simulink model "snb_bx"  (R2012b)
settings: Solver=FixedStepDiscrete  SolverMode=SingleTasking  StartTime=0.0  StopTime=10000  RelTol=1e-3
undefined symbols (not defined in the file): Down, pfb_coeff_gen_calc, Up, xlipgetpartsetting
libraries: xbsIndex_r4 x14917, casper_library_misc x20, casper_library_communications x8, xps_library x3, casper_library_delays x3
(part 50 of 96)

== system snb_bx/mix_dec_fir/mixer/dds ==
  lo_const0 : Subsystem  AncestorBlock=casper_library_downconverter/lo_const  mask(lo_const){n_bits=10, phase=0}
      mask prompts: n_bits "Output Bitwidth"; phase "Phase (0 to 2*pi)"
      mask help:
      | Generates a complex constant associated with the
      | phase supplied as a parameter.
      mask init:
      | lo_const_init(gcb, ...
      |     'n_bits', n_bits, ...
      |     'phase', phase);
      mask Help: eval('xlWeb(''http://casper.berkeley.edu/wiki/Lo_const'')')
  lo_const1 : Subsystem  AncestorBlock=casper_library_downconverter/lo_const  mask(lo_const){n_bits=10, phase=1.5708}
      mask prompts: n_bits "Output Bitwidth"; phase "Phase (0 to 2*pi)"
      mask help:
      | Generates a complex constant associated with the
      | phase supplied as a parameter.
      mask init:
      | lo_const_init(gcb, ...
      |     'n_bits', n_bits, ...
      |     'phase', phase);
      mask Help: eval('xlWeb(''http://casper.berkeley.edu/wiki/Lo_const'')')
  lo_const2 : Subsystem  AncestorBlock=casper_library_downconverter/lo_const  mask(lo_const){n_bits=10, phase=3.1416}
      mask prompts: n_bits "Output Bitwidth"; phase "Phase (0 to 2*pi)"
      mask help:
      | Generates a complex constant associated with the
      | phase supplied as a parameter.
      mask init:
      | lo_const_init(gcb, ...
      |     'n_bits', n_bits, ...
      |     'phase', phase);
      mask Help: eval('xlWeb(''http://casper.berkeley.edu/wiki/Lo_const'')')
  lo_const3 : Subsystem  AncestorBlock=casper_library_downconverter/lo_const  mask(lo_const){n_bits=10, phase=4.7124}
      mask prompts: n_bits "Output Bitwidth"; phase "Phase (0 to 2*pi)"
      mask help:
      | Generates a complex constant associated with the
      | phase supplied as a parameter.
      mask init:
      | lo_const_init(gcb, ...
      |     'n_bits', n_bits, ...
      |     'phase', phase);
      mask Help: eval('xlWeb(''http://casper.berkeley.edu/wiki/Lo_const'')')
  lo_const4 : Subsystem  AncestorBlock=casper_library_downconverter/lo_const  mask(lo_const){n_bits=10, phase=6.2832}
      mask prompts: n_bits "Output Bitwidth"; phase "Phase (0 to 2*pi)"
      mask help:
      | Generates a complex constant associated with the
      | phase supplied as a parameter.
      mask init:
      | lo_const_init(gcb, ...
      |     'n_bits', n_bits, ...
      |     'phase', phase);
      mask Help: eval('xlWeb(''http://casper.berkeley.edu/wiki/Lo_const'')')
  lo_const5 : Subsystem  AncestorBlock=casper_library_downconverter/lo_const  mask(lo_const){n_bits=10, phase=7.854}
      mask prompts: n_bits "Output Bitwidth"; phase "Phase (0 to 2*pi)"
      mask help:
      | Generates a complex constant associated with the
      | phase supplied as a parameter.
      mask init:
      | lo_const_init(gcb, ...
      |     'n_bits', n_bits, ...
      |     'phase', phase);
      mask Help: eval('xlWeb(''http://casper.berkeley.edu/wiki/Lo_const'')')
  lo_const6 : Subsystem  AncestorBlock=casper_library_downconverter/lo_const  mask(lo_const){n_bits=10, phase=9.4248}
      mask prompts: n_bits "Output Bitwidth"; phase "Phase (0 to 2*pi)"
      mask help:
      | Generates a complex constant associated with the
      | phase supplied as a parameter.
      mask init:
      | lo_const_init(gcb, ...
      |     'n_bits', n_bits, ...
      |     'phase', phase);
      mask Help: eval('xlWeb(''http://casper.berkeley.edu/wiki/Lo_const'')')
  lo_const7 : Subsystem  AncestorBlock=casper_library_downconverter/lo_const  mask(lo_const){n_bits=10, phase=10.9956}
      mask prompts: n_bits "Output Bitwidth"; phase "Phase (0 to 2*pi)"
      mask help:
      | Generates a complex constant associated with the
      | phase supplied as a parameter.
      mask init:
      | lo_const_init(gcb, ...
      |     'n_bits', n_bits, ...
      |     'phase', phase);
      mask Help: eval('xlWeb(''http://casper.berkeley.edu/wiki/Lo_const'')')
  sin0 : Outport
  cos0 : Outport  Port=2
  sin1 : Outport  Port=3
  cos1 : Outport  Port=4
  sin2 : Outport  Port=5
  cos2 : Outport  Port=6
  sin3 : Outport  Port=7
  cos3 : Outport  Port=8
  sin4 : Outport  Port=9
  cos4 : Outport  Port=10
  sin5 : Outport  Port=11
  cos5 : Outport  Port=12
  sin6 : Outport  Port=13
  cos6 : Outport  Port=14
  sin7 : Outport  Port=15
  cos7 : Outport  Port=16
  wires:
  lo_const0/1(sin) -> sin0/1
  lo_const0/2(cos) -> cos0/1
  lo_const1/1(sin) -> sin1/1
  lo_const1/2(cos) -> cos1/1
  lo_const2/1(sin) -> sin2/1
  lo_const2/2(cos) -> cos2/1
  lo_const3/1(sin) -> sin3/1
  lo_const3/2(cos) -> cos3/1
  lo_const4/1(sin) -> sin4/1
  lo_const4/2(cos) -> cos4/1
  lo_const5/1(sin) -> sin5/1
  lo_const5/2(cos) -> cos5/1
  lo_const6/1(sin) -> sin6/1
  lo_const6/2(cos) -> cos6/1
  lo_const7/1(sin) -> sin7/1
  lo_const7/2(cos) -> cos7/1

== system snb_bx/mix_dec_fir/mixer/rcmult1 ==
  d : Inport
  sin : Inport  Port=2
  cos : Inport  Port=3
  Mult0 : xbsIndex_r4/Mult  precision=Full  arith_type="Signed  (2's comp)"  n_bits=8  bin_pt=2  quantization=Truncate  overflow=Wrap  en=off  latency=latency  dbl_ovrd=off  use_behavioral_HDL=off  opt=Speed  use_embedded=on  optimum_pipeline=off  pipeline=on  use_rpm=off  placement_style=Rectangular shape  block_type=mult
  Mult1 : xbsIndex_r4/Mult  precision=Full  arith_type="Signed  (2's comp)"  n_bits=8  bin_pt=2  quantization=Truncate  overflow=Wrap  en=off  latency=latency  dbl_ovrd=off  use_behavioral_HDL=off  opt=Speed  use_embedded=on  optimum_pipeline=off  pipeline=on  use_rpm=off  placement_style=Rectangular shape  block_type=mult
  real : Outport
  imag : Outport  Port=2
  wires:
  cos/1 -> Mult0/2
  sin/1 -> Mult1/2
  d/1 -> Mult1/1, Mult0/1
  Mult0/1 -> real/1
  Mult1/1 -> imag/1

== system snb_bx/mix_dec_fir/mixer/rcmult2 ==
  d : Inport
  sin : Inport  Port=2
  cos : Inport  Port=3
  Mult0 : xbsIndex_r4/Mult  precision=Full  arith_type="Signed  (2's comp)"  n_bits=8  bin_pt=2  quantization=Truncate  overflow=Wrap  en=off  latency=latency  dbl_ovrd=off  use_behavioral_HDL=off  opt=Speed  use_embedded=on  optimum_pipeline=off  pipeline=on  use_rpm=off  placement_style=Rectangular shape  block_type=mult
  Mult1 : xbsIndex_r4/Mult  precision=Full  arith_type="Signed  (2's comp)"  n_bits=8  bin_pt=2  quantization=Truncate  overflow=Wrap  en=off  latency=latency  dbl_ovrd=off  use_behavioral_HDL=off  opt=Speed  use_embedded=on  optimum_pipeline=off  pipeline=on  use_rpm=off  placement_style=Rectangular shape  block_type=mult
  real : Outport
  imag : Outport  Port=2
  wires:
  cos/1 -> Mult0/2
  sin/1 -> Mult1/2
  d/1 -> Mult1/1, Mult0/1
  Mult0/1 -> real/1
  Mult1/1 -> imag/1

== system snb_bx/mix_dec_fir/mixer/rcmult3 ==
  d : Inport
  sin : Inport  Port=2
  cos : Inport  Port=3
  Mult0 : xbsIndex_r4/Mult  precision=Full  arith_type="Signed  (2's comp)"  n_bits=8  bin_pt=2  quantization=Truncate  overflow=Wrap  en=off  latency=latency  dbl_ovrd=off  use_behavioral_HDL=off  opt=Speed  use_embedded=on  optimum_pipeline=off  pipeline=on  use_rpm=off  placement_style=Rectangular shape  block_type=mult
  Mult1 : xbsIndex_r4/Mult  precision=Full  arith_type="Signed  (2's comp)"  n_bits=8  bin_pt=2  quantization=Truncate  overflow=Wrap  en=off  latency=latency  dbl_ovrd=off  use_behavioral_HDL=off  opt=Speed  use_embedded=on  optimum_pipeline=off  pipeline=on  use_rpm=off  placement_style=Rectangular shape  block_type=mult
  real : Outport
  imag : Outport  Port=2
  wires:
  cos/1 -> Mult0/2
  sin/1 -> Mult1/2
  d/1 -> Mult1/1, Mult0/1
  Mult0/1 -> real/1
  Mult1/1 -> imag/1

== system snb_bx/mix_dec_fir/mixer/rcmult4 ==
  d : Inport
  sin : Inport  Port=2
  cos : Inport  Port=3
  Mult0 : xbsIndex_r4/Mult  precision=Full  arith_type="Signed  (2's comp)"  n_bits=8  bin_pt=2  quantization=Truncate  overflow=Wrap  en=off  latency=latency  dbl_ovrd=off  use_behavioral_HDL=off  opt=Speed  use_embedded=on  optimum_pipeline=off  pipeline=on  use_rpm=off  placement_style=Rectangular shape  block_type=mult
  Mult1 : xbsIndex_r4/Mult  precision=Full  arith_type="Signed  (2's comp)"  n_bits=8  bin_pt=2  quantization=Truncate  overflow=Wrap  en=off  latency=latency  dbl_ovrd=off  use_behavioral_HDL=off  opt=Speed  use_embedded=on  optimum_pipeline=off  pipeline=on  use_rpm=off  placement_style=Rectangular shape  block_type=mult
  real : Outport
  imag : Outport  Port=2
  wires:
  cos/1 -> Mult0/2
  sin/1 -> Mult1/2
  d/1 -> Mult1/1, Mult0/1
  Mult0/1 -> real/1
  Mult1/1 -> imag/1

== system snb_bx/mix_dec_fir/mixer/rcmult5 ==
  d : Inport
  sin : Inport  Port=2
  cos : Inport  Port=3
  Mult0 : xbsIndex_r4/Mult  precision=Full  arith_type="Signed  (2's comp)"  n_bits=8  bin_pt=2  quantization=Truncate  overflow=Wrap  en=off  latency=latency  dbl_ovrd=off  use_behavioral_HDL=off  opt=Speed  use_embedded=on  optimum_pipeline=off  pipeline=on  use_rpm=off  placement_style=Rectangular shape  block_type=mult
  Mult1 : xbsIndex_r4/Mult  precision=Full  arith_type="Signed  (2's comp)"  n_bits=8  bin_pt=2  quantization=Truncate  overflow=Wrap  en=off  latency=latency  dbl_ovrd=off  use_behavioral_HDL=off  opt=Speed  use_embedded=on  optimum_pipeline=off  pipeline=on  use_rpm=off  placement_style=Rectangular shape  block_type=mult
  real : Outport
  imag : Outport  Port=2
  wires:
  cos/1 -> Mult0/2
  sin/1 -> Mult1/2
  d/1 -> Mult1/1, Mult0/1
  Mult0/1 -> real/1
  Mult1/1 -> imag/1

== system snb_bx/mix_dec_fir/mixer/rcmult6 ==
  d : Inport
  sin : Inport  Port=2
  cos : Inport  Port=3
  Mult0 : xbsIndex_r4/Mult  precision=Full  arith_type="Signed  (2's comp)"  n_bits=8  bin_pt=2  quantization=Truncate  overflow=Wrap  en=off  latency=latency  dbl_ovrd=off  use_behavioral_HDL=off  opt=Speed  use_embedded=on  optimum_pipeline=off  pipeline=on  use_rpm=off  placement_style=Rectangular shape  block_type=mult
  Mult1 : xbsIndex_r4/Mult  precision=Full  arith_type="Signed  (2's comp)"  n_bits=8  bin_pt=2  quantization=Truncate  overflow=Wrap  en=off  latency=latency  dbl_ovrd=off  use_behavioral_HDL=off  opt=Speed  use_embedded=on  optimum_pipeline=off  pipeline=on  use_rpm=off  placement_style=Rectangular shape  block_type=mult
  real : Outport
  imag : Outport  Port=2
  wires:
  cos/1 -> Mult0/2
  sin/1 -> Mult1/2
  d/1 -> Mult1/1, Mult0/1
  Mult0/1 -> real/1
  Mult1/1 -> imag/1

== system snb_bx/mix_dec_fir/mixer/rcmult7 ==
  d : Inport
  sin : Inport  Port=2
  cos : Inport  Port=3
  Mult0 : xbsIndex_r4/Mult  precision=Full  arith_type="Signed  (2's comp)"  n_bits=8  bin_pt=2  quantization=Truncate  overflow=Wrap  en=off  latency=latency  dbl_ovrd=off  use_behavioral_HDL=off  opt=Speed  use_embedded=on  optimum_pipeline=off  pipeline=on  use_rpm=off  placement_style=Rectangular shape  block_type=mult
  Mult1 : xbsIndex_r4/Mult  precision=Full  arith_type="Signed  (2's comp)"  n_bits=8  bin_pt=2  quantization=Truncate  overflow=Wrap  en=off  latency=latency  dbl_ovrd=off  use_behavioral_HDL=off  opt=Speed  use_embedded=on  optimum_pipeline=off  pipeline=on  use_rpm=off  placement_style=Rectangular shape  block_type=mult
  real : Outport
  imag : Outport  Port=2
  wires:
  cos/1 -> Mult0/2
  sin/1 -> Mult1/2
  d/1 -> Mult1/1, Mult0/1
  Mult0/1 -> real/1
  Mult1/1 -> imag/1

== system snb_bx/mix_dec_fir/mixer/rcmult8 ==
  d : Inport
  sin : Inport  Port=2
  cos : Inport  Port=3
  Mult0 : xbsIndex_r4/Mult  precision=Full  arith_type="Signed  (2's comp)"  n_bits=8  bin_pt=2  quantization=Truncate  overflow=Wrap  en=off  latency=latency  dbl_ovrd=off  use_behavioral_HDL=off  opt=Speed  use_embedded=on  optimum_pipeline=off  pipeline=on  use_rpm=off  placement_style=Rectangular shape  block_type=mult
  Mult1 : xbsIndex_r4/Mult  precision=Full  arith_type="Signed  (2's comp)"  n_bits=8  bin_pt=2  quantization=Truncate  overflow=Wrap  en=off  latency=latency  dbl_ovrd=off  use_behavioral_HDL=off  opt=Speed  use_embedded=on  optimum_pipeline=off  pipeline=on  use_rpm=off  placement_style=Rectangular shape  block_type=mult
  real : Outport
  imag : Outport  Port=2
  wires:
  cos/1 -> Mult0/2
  sin/1 -> Mult1/2
  d/1 -> Mult1/1, Mult0/1
  Mult0/1 -> real/1
  Mult1/1 -> imag/1

== system snb_bx/mix_dec_fir/mixer1/dds ==
  lo_const0 : Subsystem  AncestorBlock=casper_library_downconverter/lo_const  mask(lo_const){n_bits=10, phase=0}
      mask prompts: n_bits "Output Bitwidth"; phase "Phase (0 to 2*pi)"
      mask help:
      | Generates a complex constant associated with the
      | phase supplied as a parameter.
      mask init:
      | lo_const_init(gcb, ...
      |     'n_bits', n_bits, ...
      |     'phase', phase);
      mask Help: eval('xlWeb(''http://casper.berkeley.edu/wiki/Lo_const'')')
  lo_const1 : Subsystem  AncestorBlock=casper_library_downconverter/lo_const  mask(lo_const){n_bits=10, phase=1.5708}
      mask prompts: n_bits "Output Bitwidth"; phase "Phase (0 to 2*pi)"
      mask help:
      | Generates a complex constant associated with the
      | phase supplied as a parameter.
      mask init:
      | lo_const_init(gcb, ...
      |     'n_bits', n_bits, ...
      |     'phase', phase);
      mask Help: eval('xlWeb(''http://casper.berkeley.edu/wiki/Lo_const'')')
  lo_const2 : Subsystem  AncestorBlock=casper_library_downconverter/lo_const  mask(lo_const){n_bits=10, phase=3.1416}
      mask prompts: n_bits "Output Bitwidth"; phase "Phase (0 to 2*pi)"
      mask help:
      | Generates a complex constant associated with the
      | phase supplied as a parameter.
      mask init:
      | lo_const_init(gcb, ...
      |     'n_bits', n_bits, ...
      |     'phase', phase);
      mask Help: eval('xlWeb(''http://casper.berkeley.edu/wiki/Lo_const'')')
  lo_const3 : Subsystem  AncestorBlock=casper_library_downconverter/lo_const  mask(lo_const){n_bits=10, phase=4.7124}
      mask prompts: n_bits "Output Bitwidth"; phase "Phase (0 to 2*pi)"
      mask help:
      | Generates a complex constant associated with the
      | phase supplied as a parameter.
      mask init:
      | lo_const_init(gcb, ...
      |     'n_bits', n_bits, ...
      |     'phase', phase);
      mask Help: eval('xlWeb(''http://casper.berkeley.edu/wiki/Lo_const'')')
  lo_const4 : Subsystem  AncestorBlock=casper_library_downconverter/lo_const  mask(lo_const){n_bits=10, phase=6.2832}
      mask prompts: n_bits "Output Bitwidth"; phase "Phase (0 to 2*pi)"
      mask help:
      | Generates a complex constant associated with the
      | phase supplied as a parameter.
      mask init:
      | lo_const_init(gcb, ...
      |     'n_bits', n_bits, ...
      |     'phase', phase);
      mask Help: eval('xlWeb(''http://casper.berkeley.edu/wiki/Lo_const'')')
  lo_const5 : Subsystem  AncestorBlock=casper_library_downconverter/lo_const  mask(lo_const){n_bits=10, phase=7.854}
      mask prompts: n_bits "Output Bitwidth"; phase "Phase (0 to 2*pi)"
      mask help:
      | Generates a complex constant associated with the
      | phase supplied as a parameter.
      mask init:
      | lo_const_init(gcb, ...
      |     'n_bits', n_bits, ...
      |     'phase', phase);
      mask Help: eval('xlWeb(''http://casper.berkeley.edu/wiki/Lo_const'')')
  lo_const6 : Subsystem  AncestorBlock=casper_library_downconverter/lo_const  mask(lo_const){n_bits=10, phase=9.4248}
      mask prompts: n_bits "Output Bitwidth"; phase "Phase (0 to 2*pi)"
      mask help:
      | Generates a complex constant associated with the
      | phase supplied as a parameter.
      mask init:
      | lo_const_init(gcb, ...
      |     'n_bits', n_bits, ...
      |     'phase', phase);
      mask Help: eval('xlWeb(''http://casper.berkeley.edu/wiki/Lo_const'')')
  lo_const7 : Subsystem  AncestorBlock=casper_library_downconverter/lo_const  mask(lo_const){n_bits=10, phase=10.9956}
      mask prompts: n_bits "Output Bitwidth"; phase "Phase (0 to 2*pi)"
      mask help:
      | Generates a complex constant associated with the
      | phase supplied as a parameter.
      mask init:
      | lo_const_init(gcb, ...
      |     'n_bits', n_bits, ...
      |     'phase', phase);
      mask Help: eval('xlWeb(''http://casper.berkeley.edu/wiki/Lo_const'')')
  sin0 : Outport
  cos0 : Outport  Port=2
  sin1 : Outport  Port=3
  cos1 : Outport  Port=4
  sin2 : Outport  Port=5
  cos2 : Outport  Port=6
  sin3 : Outport  Port=7
  cos3 : Outport  Port=8
  sin4 : Outport  Port=9
  cos4 : Outport  Port=10
  sin5 : Outport  Port=11
  cos5 : Outport  Port=12
  sin6 : Outport  Port=13
  cos6 : Outport  Port=14
  sin7 : Outport  Port=15
  cos7 : Outport  Port=16
  wires:
  lo_const7/2(cos) -> cos7/1
  lo_const7/1(sin) -> sin7/1
  lo_const6/2(cos) -> cos6/1
  lo_const6/1(sin) -> sin6/1
  lo_const5/2(cos) -> cos5/1
  lo_const5/1(sin) -> sin5/1
  lo_const4/2(cos) -> cos4/1
  lo_const4/1(sin) -> sin4/1
  lo_const3/2(cos) -> cos3/1
  lo_const3/1(sin) -> sin3/1
  lo_const2/2(cos) -> cos2/1
  lo_const2/1(sin) -> sin2/1
  lo_const1/2(cos) -> cos1/1
  lo_const1/1(sin) -> sin1/1
  lo_const0/2(cos) -> cos0/1
  lo_const0/1(sin) -> sin0/1

== system snb_bx/mix_dec_fir/mixer1/rcmult1 ==
  d : Inport
  sin : Inport  Port=2
  cos : Inport  Port=3
  Mult0 : xbsIndex_r4/Mult  precision=Full  arith_type="Signed  (2's comp)"  n_bits=8  bin_pt=2  quantization=Truncate  overflow=Wrap  en=off  latency=latency  dbl_ovrd=off  use_behavioral_HDL=off  opt=Speed  use_embedded=on  optimum_pipeline=off  pipeline=on  use_rpm=off  placement_style=Rectangular shape  block_type=mult
  Mult1 : xbsIndex_r4/Mult  precision=Full  arith_type="Signed  (2's comp)"  n_bits=8  bin_pt=2  quantization=Truncate  overflow=Wrap  en=off  latency=latency  dbl_ovrd=off  use_behavioral_HDL=off  opt=Speed  use_embedded=on  optimum_pipeline=off  pipeline=on  use_rpm=off  placement_style=Rectangular shape  block_type=mult
  real : Outport
  imag : Outport  Port=2
  wires:
  Mult1/1 -> imag/1
  Mult0/1 -> real/1
  d/1 -> Mult0/1, Mult1/1
  sin/1 -> Mult1/2
  cos/1 -> Mult0/2

== system snb_bx/mix_dec_fir/mixer1/rcmult2 ==
  d : Inport
  sin : Inport  Port=2
  cos : Inport  Port=3
  Mult0 : xbsIndex_r4/Mult  precision=Full  arith_type="Signed  (2's comp)"  n_bits=8  bin_pt=2  quantization=Truncate  overflow=Wrap  en=off  latency=latency  dbl_ovrd=off  use_behavioral_HDL=off  opt=Speed  use_embedded=on  optimum_pipeline=off  pipeline=on  use_rpm=off  placement_style=Rectangular shape  block_type=mult
  Mult1 : xbsIndex_r4/Mult  precision=Full  arith_type="Signed  (2's comp)"  n_bits=8  bin_pt=2  quantization=Truncate  overflow=Wrap  en=off  latency=latency  dbl_ovrd=off  use_behavioral_HDL=off  opt=Speed  use_embedded=on  optimum_pipeline=off  pipeline=on  use_rpm=off  placement_style=Rectangular shape  block_type=mult
  real : Outport
  imag : Outport  Port=2
  wires:
  Mult1/1 -> imag/1
  Mult0/1 -> real/1
  d/1 -> Mult0/1, Mult1/1
  sin/1 -> Mult1/2
  cos/1 -> Mult0/2

== system snb_bx/mix_dec_fir/mixer1/rcmult3 ==
  d : Inport
  sin : Inport  Port=2
  cos : Inport  Port=3
  Mult0 : xbsIndex_r4/Mult  precision=Full  arith_type="Signed  (2's comp)"  n_bits=8  bin_pt=2  quantization=Truncate  overflow=Wrap  en=off  latency=latency  dbl_ovrd=off  use_behavioral_HDL=off  opt=Speed  use_embedded=on  optimum_pipeline=off  pipeline=on  use_rpm=off  placement_style=Rectangular shape  block_type=mult
  Mult1 : xbsIndex_r4/Mult  precision=Full  arith_type="Signed  (2's comp)"  n_bits=8  bin_pt=2  quantization=Truncate  overflow=Wrap  en=off  latency=latency  dbl_ovrd=off  use_behavioral_HDL=off  opt=Speed  use_embedded=on  optimum_pipeline=off  pipeline=on  use_rpm=off  placement_style=Rectangular shape  block_type=mult
  real : Outport
  imag : Outport  Port=2
  wires:
  Mult1/1 -> imag/1
  Mult0/1 -> real/1
  d/1 -> Mult0/1, Mult1/1
  sin/1 -> Mult1/2
  cos/1 -> Mult0/2

== system snb_bx/mix_dec_fir/mixer1/rcmult4 ==
  d : Inport
  sin : Inport  Port=2
  cos : Inport  Port=3
  Mult0 : xbsIndex_r4/Mult  precision=Full  arith_type="Signed  (2's comp)"  n_bits=8  bin_pt=2  quantization=Truncate  overflow=Wrap  en=off  latency=latency  dbl_ovrd=off  use_behavioral_HDL=off  opt=Speed  use_embedded=on  optimum_pipeline=off  pipeline=on  use_rpm=off  placement_style=Rectangular shape  block_type=mult
  Mult1 : xbsIndex_r4/Mult  precision=Full  arith_type="Signed  (2's comp)"  n_bits=8  bin_pt=2  quantization=Truncate  overflow=Wrap  en=off  latency=latency  dbl_ovrd=off  use_behavioral_HDL=off  opt=Speed  use_embedded=on  optimum_pipeline=off  pipeline=on  use_rpm=off  placement_style=Rectangular shape  block_type=mult
  real : Outport
  imag : Outport  Port=2
  wires:
  Mult1/1 -> imag/1
  Mult0/1 -> real/1
  d/1 -> Mult0/1, Mult1/1
  sin/1 -> Mult1/2
  cos/1 -> Mult0/2

== system snb_bx/mix_dec_fir/mixer1/rcmult5 ==
  d : Inport
  sin : Inport  Port=2
  cos : Inport  Port=3
  Mult0 : xbsIndex_r4/Mult  precision=Full  arith_type="Signed  (2's comp)"  n_bits=8  bin_pt=2  quantization=Truncate  overflow=Wrap  en=off  latency=latency  dbl_ovrd=off  use_behavioral_HDL=off  opt=Speed  use_embedded=on  optimum_pipeline=off  pipeline=on  use_rpm=off  placement_style=Rectangular shape  block_type=mult
  Mult1 : xbsIndex_r4/Mult  precision=Full  arith_type="Signed  (2's comp)"  n_bits=8  bin_pt=2  quantization=Truncate  overflow=Wrap  en=off  latency=latency  dbl_ovrd=off  use_behavioral_HDL=off  opt=Speed  use_embedded=on  optimum_pipeline=off  pipeline=on  use_rpm=off  placement_style=Rectangular shape  block_type=mult
  real : Outport
  imag : Outport  Port=2
  wires:
  Mult1/1 -> imag/1
  Mult0/1 -> real/1
  d/1 -> Mult0/1, Mult1/1
  sin/1 -> Mult1/2
  cos/1 -> Mult0/2

== system snb_bx/mix_dec_fir/mixer1/rcmult6 ==
  d : Inport
  sin : Inport  Port=2
  cos : Inport  Port=3
  Mult0 : xbsIndex_r4/Mult  precision=Full  arith_type="Signed  (2's comp)"  n_bits=8  bin_pt=2  quantization=Truncate  overflow=Wrap  en=off  latency=latency  dbl_ovrd=off  use_behavioral_HDL=off  opt=Speed  use_embedded=on  optimum_pipeline=off  pipeline=on  use_rpm=off  placement_style=Rectangular shape  block_type=mult
  Mult1 : xbsIndex_r4/Mult  precision=Full  arith_type="Signed  (2's comp)"  n_bits=8  bin_pt=2  quantization=Truncate  overflow=Wrap  en=off  latency=latency  dbl_ovrd=off  use_behavioral_HDL=off  opt=Speed  use_embedded=on  optimum_pipeline=off  pipeline=on  use_rpm=off  placement_style=Rectangular shape  block_type=mult
  real : Outport
  imag : Outport  Port=2
  wires:
  Mult1/1 -> imag/1
  Mult0/1 -> real/1
  d/1 -> Mult0/1, Mult1/1
  sin/1 -> Mult1/2
  cos/1 -> Mult0/2

== system snb_bx/mix_dec_fir/mixer1/rcmult7 ==
  d : Inport
  sin : Inport  Port=2
  cos : Inport  Port=3
  Mult0 : xbsIndex_r4/Mult  precision=Full  arith_type="Signed  (2's comp)"  n_bits=8  bin_pt=2  quantization=Truncate  overflow=Wrap  en=off  latency=latency  dbl_ovrd=off  use_behavioral_HDL=off  opt=Speed  use_embedded=on  optimum_pipeline=off  pipeline=on  use_rpm=off  placement_style=Rectangular shape  block_type=mult
  Mult1 : xbsIndex_r4/Mult  precision=Full  arith_type="Signed  (2's comp)"  n_bits=8  bin_pt=2  quantization=Truncate  overflow=Wrap  en=off  latency=latency  dbl_ovrd=off  use_behavioral_HDL=off  opt=Speed  use_embedded=on  optimum_pipeline=off  pipeline=on  use_rpm=off  placement_style=Rectangular shape  block_type=mult
  real : Outport
  imag : Outport  Port=2
  wires:
  Mult1/1 -> imag/1
  Mult0/1 -> real/1
  d/1 -> Mult0/1, Mult1/1
  sin/1 -> Mult1/2
  cos/1 -> Mult0/2

== system snb_bx/mix_dec_fir/mixer1/rcmult8 ==
  d : Inport
  sin : Inport  Port=2
  cos : Inport  Port=3
  Mult0 : xbsIndex_r4/Mult  precision=Full  arith_type="Signed  (2's comp)"  n_bits=8  bin_pt=2  quantization=Truncate  overflow=Wrap  en=off  latency=latency  dbl_ovrd=off  use_behavioral_HDL=off  opt=Speed  use_embedded=on  optimum_pipeline=off  pipeline=on  use_rpm=off  placement_style=Rectangular shape  block_type=mult
  Mult1 : xbsIndex_r4/Mult  precision=Full  arith_type="Signed  (2's comp)"  n_bits=8  bin_pt=2  quantization=Truncate  overflow=Wrap  en=off  latency=latency  dbl_ovrd=off  use_behavioral_HDL=off  opt=Speed  use_embedded=on  optimum_pipeline=off  pipeline=on  use_rpm=off  placement_style=Rectangular shape  block_type=mult
  real : Outport
  imag : Outport  Port=2
  wires:
  Mult1/1 -> imag/1
  Mult0/1 -> real/1
  d/1 -> Mult0/1, Mult1/1
  sin/1 -> Mult1/2
  cos/1 -> Mult0/2

== system snb_bx/pack/spead_pack/edge_detect1 ==
  in : Inport
  Delay : xbsIndex_r4/Delay  rst=off  infoeditControl=Selection of Reset will increase slice count due to use of real FFs and instead of SRLs  en=off  latency=1  dbl_ovrd=off  reg_retiming=off  block_type=delay
      settings: xl_area=[0, 0, 0, 0, 0, 0, 0]
  Inverter : xbsIndex_r4/Inverter  en=off  latency=0  dbl_ovrd=off  block_type=inv
      settings: xl_area=[0, 0, 0, 0, 0, 0, 0]
  edge_op : xbsIndex_r4/Logical  logical_function=NOR  inputs=2  en=off  latency=0  precision=Full  arith_type=Unsigned  n_bits=8  bin_pt=2  align_bp=on  dbl_ovrd=off  block_type=logical
      settings: xl_area=[0, 0, 0, 0, 0, 0, 0]
  out : Outport
  wires:
  Delay/1 -> edge_op/2
  in/1 -> Delay/1, Inverter/1
  edge_op/1 -> out/1
  Inverter/1 -> edge_op/1

== system snb_bx/pack/spead_pack/edge_detect2 ==
  in : Inport
  Delay : xbsIndex_r4/Delay  rst=off  infoeditControl=Selection of Reset will increase slice count due to use of real FFs and instead of SRLs  en=off  latency=1  dbl_ovrd=off  reg_retiming=off  block_type=delay
      settings: xl_area=[0, 0, 0, 0, 0, 0, 0]
  Inverter : xbsIndex_r4/Inverter  en=off  latency=0  dbl_ovrd=off  block_type=inv
      settings: xl_area=[0, 0, 0, 0, 0, 0, 0]
  edge_op : xbsIndex_r4/Logical  logical_function=NOR  inputs=2  en=off  latency=0  precision=Full  arith_type=Unsigned  n_bits=8  bin_pt=2  align_bp=on  dbl_ovrd=off  block_type=logical
      settings: xl_area=[0, 0, 0, 0, 0, 0, 0]
  out : Outport
  wires:
  Inverter/1 -> edge_op/1
  edge_op/1 -> out/1
  in/1 -> Inverter/1, Delay/1
  Delay/1 -> edge_op/2

== system snb_bx/pack/spead_pack1/edge_detect1 ==
  in : Inport
  Delay : xbsIndex_r4/Delay  rst=off  infoeditControl=Selection of Reset will increase slice count due to use of real FFs and instead of SRLs  en=off  latency=1  dbl_ovrd=off  reg_retiming=off  block_type=delay
      settings: xl_area=[0, 0, 0, 0, 0, 0, 0]
  Inverter : xbsIndex_r4/Inverter  en=off  latency=0  dbl_ovrd=off  block_type=inv
      settings: xl_area=[0, 0, 0, 0, 0, 0, 0]
  edge_op : xbsIndex_r4/Logical  logical_function=NOR  inputs=2  en=off  latency=0  precision=Full  arith_type=Unsigned  n_bits=8  bin_pt=2  align_bp=on  dbl_ovrd=off  block_type=logical
      settings: xl_area=[0, 0, 0, 0, 0, 0, 0]
  out : Outport
  wires:
  Inverter/1 -> edge_op/1
  edge_op/1 -> out/1
  in/1 -> Inverter/1, Delay/1
  Delay/1 -> edge_op/2

== system snb_bx/pack/spead_pack1/edge_detect2 ==
  in : Inport
  Delay : xbsIndex_r4/Delay  rst=off  infoeditControl=Selection of Reset will increase slice count due to use of real FFs and instead of SRLs  en=off  latency=1  dbl_ovrd=off  reg_retiming=off  block_type=delay
      settings: xl_area=[0, 0, 0, 0, 0, 0, 0]
  Inverter : xbsIndex_r4/Inverter  en=off  latency=0  dbl_ovrd=off  block_type=inv
      settings: xl_area=[0, 0, 0, 0, 0, 0, 0]
  edge_op : xbsIndex_r4/Logical  logical_function=NOR  inputs=2  en=off  latency=0  precision=Full  arith_type=Unsigned  n_bits=8  bin_pt=2  align_bp=on  dbl_ovrd=off  block_type=logical
      settings: xl_area=[0, 0, 0, 0, 0, 0, 0]
  out : Outport
  wires:
  Delay/1 -> edge_op/2
  in/1 -> Delay/1, Inverter/1
  edge_op/1 -> out/1
  Inverter/1 -> edge_op/1

== system snb_bx/pack/spead_pack2/edge_detect1 ==
  in : Inport
  Delay : xbsIndex_r4/Delay  rst=off  infoeditControl=Selection of Reset will increase slice count due to use of real FFs and instead of SRLs  en=off  latency=1  dbl_ovrd=off  reg_retiming=off  block_type=delay
      settings: xl_area=[0, 0, 0, 0, 0, 0, 0]
  Inverter : xbsIndex_r4/Inverter  en=off  latency=0  dbl_ovrd=off  block_type=inv
      settings: xl_area=[0, 0, 0, 0, 0, 0, 0]
  edge_op : xbsIndex_r4/Logical  logical_function=NOR  inputs=2  en=off  latency=0  precision=Full  arith_type=Unsigned  n_bits=8  bin_pt=2  align_bp=on  dbl_ovrd=off  block_type=logical
      settings: xl_area=[0, 0, 0, 0, 0, 0, 0]
  out : Outport
  wires:
  Delay/1 -> edge_op/2
  in/1 -> Delay/1, Inverter/1
  edge_op/1 -> out/1
  Inverter/1 -> edge_op/1

== system snb_bx/pack/spead_pack2/edge_detect2 ==
  in : Inport
  Delay : xbsIndex_r4/Delay  rst=off  infoeditControl=Selection of Reset will increase slice count due to use of real FFs and instead of SRLs  en=off  latency=1  dbl_ovrd=off  reg_retiming=off  block_type=delay
      settings: xl_area=[0, 0, 0, 0, 0, 0, 0]
  Inverter : xbsIndex_r4/Inverter  en=off  latency=0  dbl_ovrd=off  block_type=inv
      settings: xl_area=[0, 0, 0, 0, 0, 0, 0]
  edge_op : xbsIndex_r4/Logical  logical_function=NOR  inputs=2  en=off  latency=0  precision=Full  arith_type=Unsigned  n_bits=8  bin_pt=2  align_bp=on  dbl_ovrd=off  block_type=logical
      settings: xl_area=[0, 0, 0, 0, 0, 0, 0]
  out : Outport
  wires:
  Inverter/1 -> edge_op/1
  edge_op/1 -> out/1
  in/1 -> Inverter/1, Delay/1
  Delay/1 -> edge_op/2

== system snb_bx/pack/spead_pack3/edge_detect1 ==
  in : Inport
  Delay : xbsIndex_r4/Delay  rst=off  infoeditControl=Selection of Reset will increase slice count due to use of real FFs and instead of SRLs  en=off  latency=1  dbl_ovrd=off  reg_retiming=off  block_type=delay
      settings: xl_area=[0, 0, 0, 0, 0, 0, 0]
  Inverter : xbsIndex_r4/Inverter  en=off  latency=0  dbl_ovrd=off  block_type=inv
      settings: xl_area=[0, 0, 0, 0, 0, 0, 0]
  edge_op : xbsIndex_r4/Logical  logical_function=NOR  inputs=2  en=off  latency=0  precision=Full  arith_type=Unsigned  n_bits=8  bin_pt=2  align_bp=on  dbl_ovrd=off  block_type=logical
      settings: xl_area=[0, 0, 0, 0, 0, 0, 0]
  out : Outport
  wires:
  Inverter/1 -> edge_op/1
  edge_op/1 -> out/1
  in/1 -> Inverter/1, Delay/1
  Delay/1 -> edge_op/2

== system snb_bx/pack/spead_pack3/edge_detect2 ==
  in : Inport
  Delay : xbsIndex_r4/Delay  rst=off  infoeditControl=Selection of Reset will increase slice count due to use of real FFs and instead of SRLs  en=off  latency=1  dbl_ovrd=off  reg_retiming=off  block_type=delay
      settings: xl_area=[0, 0, 0, 0, 0, 0, 0]
  Inverter : xbsIndex_r4/Inverter  en=off  latency=0  dbl_ovrd=off  block_type=inv
      settings: xl_area=[0, 0, 0, 0, 0, 0, 0]
  edge_op : xbsIndex_r4/Logical  logical_function=NOR  inputs=2  en=off  latency=0  precision=Full  arith_type=Unsigned  n_bits=8  bin_pt=2  align_bp=on  dbl_ovrd=off  block_type=logical
      settings: xl_area=[0, 0, 0, 0, 0, 0, 0]
  out : Outport
  wires:
  Delay/1 -> edge_op/2
  in/1 -> Delay/1, Inverter/1
  edge_op/1 -> out/1
  Inverter/1 -> edge_op/1

== system snb_bx/pfb_fft/pfb_fir_generic/bus_convert ==
  din : Inport
  bussify : Subsystem  AncestorBlock=casper_library_flow_control/bus_create  mask(bus_create){inputNum=4}
      mask prompts: inputNum "Number of inputs:"
      mask init:
      | bus_create_init(gcb,...
      |     'inputNum', inputNum);
  conv1 : Subsystem  AncestorBlock=casper_library_misc/convert  mask(convert){bin_pt_in=35, n_bits_out=18, bin_pt_out=17, quantization=Round  (unbiased: Even Values), overflow=Wrap, latency=2}
      mask prompts: bin_pt_in "Binary Point In"; n_bits_out "Bit Width Out"; bin_pt_out "Binary Point Out"
      mask help:
      | Convert input value to the specified bit width and precision.
      |
      | Does not support upscaling number of fractional bits (eg 8_5 to 8_4 is ok, but not 8_4 to 8_5).
      mask init:
      | convert_init(gcb, ...
      |     'bin_pt_in',bin_pt_in, ...
      |     'n_bits_out',n_bits_out,...
      |     'bin_pt_out',bin_pt_out, ...
      |     'quantization',quantization,...
      |     'overflow',overflow,...
      |     'latency',latency);
      settings: AttributesFormatString=|
      | N_35 ==> 18_17
      | round even, wrap
      | latency = 2
      mask Help:
      | <pre>
      | Description::
      | 
      | Outputs converted version of the input.
      | 
      | Mask Parameters::
      | 
      | Binary Point In (bin_pt_in): Specifies the binary point location in the input.
      | 
      | Bit Width Out (n_bits_out): Specifies the width of the output.
      | 
      | Binary Point Out (bin_pt_out): Specifies the binary point location in the output.
      | 
      | Quantization (quantization): Specifies quantization handling.
      | 
      | Overflow (overflow): Specifies overflow handling.
      | 
      | Latency (latency): Specifies the latency of the underlying adder block, which is the overall
      | latency of this block as well.
      | </pre>
      mask TypeOptions quantization: Truncate | Round  (unbiased: +/- Inf) | Round  (unbiased: Even Values) | Round  (unbiased: Zero) | Round  (unbiased: Odd Values) | Round  (biased: Up) | Round  (biased: Down)
      mask TypeOptions overflow: Wrap | Saturate | Error
  conv2 : Subsystem  AncestorBlock=casper_library_misc/convert  mask(convert){bin_pt_in=35, n_bits_out=18, bin_pt_out=17, quantization=Round  (unbiased: Even Values), overflow=Wrap, latency=2}
      mask prompts: bin_pt_in "Binary Point In"; n_bits_out "Bit Width Out"; bin_pt_out "Binary Point Out"
      mask help:
      | Convert input value to the specified bit width and precision.
      |
      | Does not support upscaling number of fractional bits (eg 8_5 to 8_4 is ok, but not 8_4 to 8_5).
      mask init: same as snb_bx/pfb_fft/pfb_fir_generic/bus_convert/conv1
      settings: AttributesFormatString=|
      | N_35 ==> 18_17
      | round even, wrap
      | latency = 2
      mask Help:
      | <pre>
      | Description::
      | 
      | Outputs converted version of the input.
      | 
      | Mask Parameters::
      | 
      | Binary Point In (bin_pt_in): Specifies the binary point location in the input.
      | 
      | Bit Width Out (n_bits_out): Specifies the width of the output.
      | 
      | Binary Point Out (bin_pt_out): Specifies the binary point location in the output.
      | 
      | Quantization (quantization): Specifies quantization handling.
      | 
      | Overflow (overflow): Specifies overflow handling.
      | 
      | Latency (latency): Specifies the latency of the underlying adder block, which is the overall
      | latency of this block as well.
      | </pre>
      mask TypeOptions quantization: Truncate | Round  (unbiased: +/- Inf) | Round  (unbiased: Even Values) | Round  (unbiased: Zero) | Round  (unbiased: Odd Values) | Round  (biased: Up) | Round  (biased: Down)
      mask TypeOptions overflow: Wrap | Saturate | Error
  conv3 : Subsystem  AncestorBlock=casper_library_misc/convert  mask(convert){bin_pt_in=35, n_bits_out=18, bin_pt_out=17, quantization=Round  (unbiased: Even Values), overflow=Wrap, latency=2}
      mask prompts: bin_pt_in "Binary Point In"; n_bits_out "Bit Width Out"; bin_pt_out "Binary Point Out"
      mask help:
      | Convert input value to the specified bit width and precision.
      |
      | Does not support upscaling number of fractional bits (eg 8_5 to 8_4 is ok, but not 8_4 to 8_5).
      mask init: same as snb_bx/pfb_fft/pfb_fir_generic/bus_convert/conv1
      settings: AttributesFormatString=|
      | N_35 ==> 18_17
      | round even, wrap
      | latency = 2
      mask Help:
      | <pre>
      | Description::
      | 
      | Outputs converted version of the input.
      | 
      | Mask Parameters::
      | 
      | Binary Point In (bin_pt_in): Specifies the binary point location in the input.
      | 
      | Bit Width Out (n_bits_out): Specifies the width of the output.
      | 
      | Binary Point Out (bin_pt_out): Specifies the binary point location in the output.
      | 
      | Quantization (quantization): Specifies quantization handling.
      | 
      | Overflow (overflow): Specifies overflow handling.
      | 
      | Latency (latency): Specifies the latency of the underlying adder block, which is the overall
      | latency of this block as well.
      | </pre>
      mask TypeOptions quantization: Truncate | Round  (unbiased: +/- Inf) | Round  (unbiased: Even Values) | Round  (unbiased: Zero) | Round  (unbiased: Odd Values) | Round  (biased: Up) | Round  (biased: Down)
      mask TypeOptions overflow: Wrap | Saturate | Error
  conv4 : Subsystem  AncestorBlock=casper_library_misc/convert  mask(convert){bin_pt_in=35, n_bits_out=18, bin_pt_out=17, quantization=Round  (unbiased: Even Values), overflow=Wrap, latency=2}
      mask prompts: bin_pt_in "Binary Point In"; n_bits_out "Bit Width Out"; bin_pt_out "Binary Point Out"
      mask help:
      | Convert input value to the specified bit width and precision.
      |
      | Does not support upscaling number of fractional bits (eg 8_5 to 8_4 is ok, but not 8_4 to 8_5).
      mask init: same as snb_bx/pfb_fft/pfb_fir_generic/bus_convert/conv1
      settings: AttributesFormatString=|
      | N_35 ==> 18_17
      | round even, wrap
      | latency = 2
      mask Help:
      | <pre>
      | Description::
      | 
      | Outputs converted version of the input.
      | 
      | Mask Parameters::
      | 
      | Binary Point In (bin_pt_in): Specifies the binary point location in the input.
      | 
      | Bit Width Out (n_bits_out): Specifies the width of the output.
      | 
      | Binary Point Out (bin_pt_out): Specifies the binary point location in the output.
      | 
      | Quantization (quantization): Specifies quantization handling.
      | 
      | Overflow (overflow): Specifies overflow handling.
      | 
      | Latency (latency): Specifies the latency of the underlying adder block, which is the overall
      | latency of this block as well.
      | </pre>
      mask TypeOptions quantization: Truncate | Round  (unbiased: +/- Inf) | Round  (unbiased: Even Values) | Round  (unbiased: Zero) | Round  (unbiased: Odd Values) | Round  (biased: Up) | Round  (biased: Down)
      mask TypeOptions overflow: Wrap | Saturate | Error
  debus : Subsystem  AncestorBlock=casper_library_flow_control/bus_expand  mask(bus_expand){mode=divisions of arbitrary size, outputNum=1, outputWidth=[43 43 43 43], outputBinaryPt=[35 35 35 35], outputArithmeticType=[1 1 1 1], show_format=on, outputToWorkspace=off, variablePrefix=, outputToModelAsWell=on}
      mask prompts: outputNum "Number of outputs:"; outputWidth "Output width [msb ... lsb]:"; outputBinaryPt "Output binary point position [msb ... lsb]:"; outputArithmeticType "Output arithmetic type (ufix=0, fix=1, bool=2) [msb ... lsb]:"; show_format "Print format string?"; outputToWorkspace "Output to workspace?"; variablePrefix "Variable name prefix:"; outputToModelAsWell "Output to model as well?"
      mask help:
      | Expands a 'bus' made using a bus_create or Xilinx
      | concat block.
      | The input will be divided into the specified number
      | of outputs with the specified arithmetic types.
      | Divisions are made from most significant bit.
      mask init: same as snb_bx/bus_expand10
      settings: AttributesFormatString=4 outputs: f43.35,f43.35,f43.35,f43.35,
      mask TypeOptions mode: divisions of equal size | divisions of arbitrary size
      mask Callback mode: bus_expand_callback();
      mask Callback outputWidth: bus_expand_callback();
      mask Callback outputToWorkspace: bus_expand_callback();
  dout : Outport
  wires:
  bussify/1(bus_out) -> dout/1
  conv4/1(out) -> bussify/4(in4)
  conv3/1(out) -> bussify/3(in3)
  conv2/1(out) -> bussify/2(in2)
  conv1/1(out) -> bussify/1(in1)
  debus/4(lsb_out1) -> conv4/1(in)
  debus/3(out2) -> conv3/1(in)
  debus/2(out3) -> conv2/1(in)
  debus/1(msb_out4) -> conv1/1(in)
  din/1 -> debus/1(bus_in)

== system snb_bx/pfb_fft/pfb_fir_generic/bus_create ==
  in1 : Inport
  in2 : Inport  Port=2
  concatenate : xbsIndex_r4/Concat  num_inputs=2  dbl_ovrd=off  block_type=concat
  reinterpret1 : xbsIndex_r4/Reinterpret  force_arith_type=on  arith_type=Unsigned  force_bin_pt=on  bin_pt=0  block_type=reinterpret
      settings: infoedit="Changes signal type without altering the binary representation.   You can changed the signal between signed and unsigned, and relocate the binary point.<br><br>Hardware notes: In hardware this block costs nothing.<br><br>Example:  Suppose the input is 6 bits wide, signed, with 2 fractional bits, and the output is forced to unsigned with 0 fractional bits.  Then an input of -2.0 (1110.00 in binary 2's complement) becomes an output of 56 (111000 in binary)."
  reinterpret2 : xbsIndex_r4/Reinterpret  force_arith_type=on  arith_type=Unsigned  force_bin_pt=on  bin_pt=0  block_type=reinterpret
      settings: infoedit="Changes signal type without altering the binary representation.   You can changed the signal between signed and unsigned, and relocate the binary point.<br><br>Hardware notes: In hardware this block costs nothing.<br><br>Example:  Suppose the input is 6 bits wide, signed, with 2 fractional bits, and the output is forced to unsigned with 0 fractional bits.  Then an input of -2.0 (1110.00 in binary 2's complement) becomes an output of 56 (111000 in binary)."
  bus_out : Outport
  wires:
  reinterpret2/1 -> concatenate/2
  in2/1 -> reinterpret2/1
  reinterpret1/1 -> concatenate/1
  in1/1 -> reinterpret1/1
  concatenate/1 -> bus_out/1

== system snb_bx/pfb_fft/pfb_fir_generic/bus_expand ==
  bus_in : Inport
  reinterpret1 : xbsIndex_r4/Reinterpret  force_arith_type=on  arith_type=Unsigned  force_bin_pt=on  bin_pt=0  block_type=reinterpret
  reinterpret2 : xbsIndex_r4/Reinterpret  force_arith_type=on  arith_type=Unsigned  force_bin_pt=on  bin_pt=0  block_type=reinterpret
  slice1 : xbsIndex_r4/Slice  nbits=36  boolean_output=off  mode=Upper Bit Location + Width  bit1=-36  base1=MSB of Input  bit0=0  base0=LSB of Input  dbl_ovrd=off  block_type=slice
  slice2 : xbsIndex_r4/Slice  nbits=36  boolean_output=off  mode=Upper Bit Location + Width  bit1=0  base1=MSB of Input  bit0=0  base0=LSB of Input  dbl_ovrd=off  block_type=slice
  msb_out2 : Outport
  lsb_out1 : Outport  Port=2
  wires:
  reinterpret1/1 -> lsb_out1/1
  slice1/1 -> reinterpret1/1
  reinterpret2/1 -> msb_out2/1
  slice2/1 -> reinterpret2/1
  bus_in/1 -> slice1/1, slice2/1

== system snb_bx/pfb_fft/pfb_fir_generic/bus_scale ==
  din : Inport
  bussify : Subsystem  AncestorBlock=casper_library_flow_control/bus_create  mask(bus_create){inputNum=4}
      mask prompts: inputNum "Number of inputs:"
      mask init:
      | bus_create_init(gcb,...
      |     'inputNum', inputNum);
  debus : Subsystem  AncestorBlock=casper_library_flow_control/bus_expand  mask(bus_expand){mode=divisions of arbitrary size, outputNum=1, outputWidth=[43 43 43 43], outputBinaryPt=[34 34 34 34], outputArithmeticType=[1 1 1 1], show_format=on, outputToWorkspace=off, variablePrefix=, outputToModelAsWell=on}
      mask prompts: outputNum "Number of outputs:"; outputWidth "Output width [msb ... lsb]:"; outputBinaryPt "Output binary point position [msb ... lsb]:"; outputArithmeticType "Output arithmetic type (ufix=0, fix=1, bool=2) [msb ... lsb]:"; show_format "Print format string?"; outputToWorkspace "Output to workspace?"; variablePrefix "Variable name prefix:"; outputToModelAsWell "Output to model as well?"
      mask help:
      | Expands a 'bus' made using a bus_create or Xilinx
      | concat block.
      | The input will be divided into the specified number
      | of outputs with the specified arithmetic types.
      | Divisions are made from most significant bit.
      mask init: same as snb_bx/bus_expand10
      settings: AttributesFormatString=4 outputs: f43.34,f43.34,f43.34,f43.34,
      mask TypeOptions mode: divisions of equal size | divisions of arbitrary size
      mask Callback mode: bus_expand_callback();
      mask Callback outputWidth: bus_expand_callback();
      mask Callback outputToWorkspace: bus_expand_callback();
  scale{1..4} (4 alike) : xbsIndex_r4/Scale  scale_factor=-1  dbl_ovrd=off  block_type=scale
  dout : Outport
  wires:
  bussify/1(bus_out) -> dout/1
  scale4/1 -> bussify/4(in4)
  scale3/1 -> bussify/3(in3)
  scale2/1 -> bussify/2(in2)
  scale1/1 -> bussify/1(in1)
  debus/4(lsb_out1) -> scale4/1
  debus/3(out2) -> scale3/1
  debus/2(out3) -> scale2/1
  debus/1(msb_out4) -> scale1/1
  din/1 -> debus/1(bus_in)

== system snb_bx/pfb_fft/pfb_fir_generic/coeff_munge ==
  din : Inport
  join : Subsystem  AncestorBlock=casper_library_flow_control/bus_create  mask(bus_create){inputNum=32}
      mask prompts: inputNum "Number of inputs:"
      mask init:
      | bus_create_init(gcb,...
      |     'inputNum', inputNum);
  reinterpret : xbsIndex_r4/Reinterpret  force_arith_type=on  arith_type=Unsigned  force_bin_pt=on  bin_pt=0  block_type=reinterpret
  reinterpret_out : xbsIndex_r4/Reinterpret  force_arith_type=on  arith_type=Unsigned  force_bin_pt=on  bin_pt=0  block_type=reinterpret
  split : Subsystem  AncestorBlock=casper_library_flow_control/bus_expand  mask(bus_expand){mode=divisions of arbitrary size, outputNum=1, outputWidth=[18 18 18 18 18 18 18 18], outputBinaryPt=[0 0 0 0 0 0 0 0], outputArithmeticType=[0 0 0 0 0 0 0 0], show_format=off, outputToWorkspace=off, variablePrefix=out, outputToModelAsWell=on}
      mask prompts: outputNum "Number of outputs:"; outputWidth "Output width [msb ... lsb]:"; outputBinaryPt "Output binary point position [msb ... lsb]:"; outputArithmeticType "Output arithmetic type (ufix=0, fix=1, bool=2) [msb ... lsb]:"; show_format "Print format string?"; outputToWorkspace "Output to workspace?"; variablePrefix "Variable name prefix:"; outputToModelAsWell "Output to model as well?"
      mask help:
      | Expands a 'bus' made using a bus_create or Xilinx
      | concat block.
      | The input will be divided into the specified number
      | of outputs with the specified arithmetic types.
      | Divisions are made from most significant bit.
      mask init: same as snb_bx/bus_expand10
      settings: AttributesFormatString=8 outputs
      mask TypeOptions mode: divisions of equal size | divisions of arbitrary size
      mask Callback mode: bus_expand_callback();
      mask Callback outputWidth: bus_expand_callback();
      mask Callback outputToWorkspace: bus_expand_callback();
  dout : Outport
  wires:
  split/1(msb_out8) -> join/32(in32), join/31(in31), join/30(in30), join/29(in29)
  split/2(out7) -> join/28(in28), join/27(in27), join/26(in26), join/25(in25)
  split/3(out6) -> join/24(in24), join/23(in23), join/22(in22), join/21(in21)
  split/4(out5) -> join/20(in20), join/19(in19), join/18(in18), join/17(in17)
  split/5(out4) -> join/16(in16), join/15(in15), join/14(in14), join/13(in13)
  split/6(out3) -> join/12(in12), join/11(in11), join/10(in10), join/9(in9)
  split/7(out2) -> join/8(in8), join/7(in7), join/6(in6), join/5(in5)
  split/8(lsb_out1) -> join/4(in4), join/3(in3), join/2(in2), join/1(in1)
  join/1(bus_out) -> reinterpret_out/1
  reinterpret/1 -> split/1(bus_in)
  din/1 -> reinterpret/1
  reinterpret_out/1 -> dout/1
